simulink model "System_Template"  (R2021b)
settings: Solver=FixedStepDiscrete  StartTime=0.0  StopTime=0.001  FixedStep=1/312.5e6  RelTol=1e-3
undefined symbols (not defined in the file or in its folder): sigbuilder_block
settings Model: DataTypeOverride=Off  Creator=max_d  LastModifiedBy=max_d
settings SolverCC: AlgebraicLoopSolver=TrustRegion
settings DataIOCC: LimitDataPoints=on  SaveOutput=off  SaveTime=off
settings OptimizationCC: BlockReduction=off  ConditionallyExecuteInputs=off  DefaultParameterBehavior=Inlined  LifeSpan=inf
settings DebuggingCC: AlgebraicLoopMsg=error  SingleTaskRateTransMsg=error  AllowSymbolicDim=off  StrictBusMsg=ErrorOnBusTreatedAsVector  SFUnexpectedBacktrackingDiag=warning  SFNoUnconditionalDefaultTransitionDiag=warning  SFExecutionAtInitializationDiag=none  SFMachineParentedDataDiag=warning  ArithmeticOperatorsInVariantConditions=warning
settings HardwareCC: ProdBitPerPointer=32  ProdBitPerSizeT=32  ProdBitPerPtrDiffT=32  ProdLargestAtomicFloat=None  ProdIntDivRoundTo=Undefined  ProdEndianess=Unspecified  ProdWordSize=32  ProdHWDeviceType=ASIC/FPGA->ASIC/FPGA  ProdEqTarget=off
settings SFSimCC: SimUseLocalCustomCode=off  CustomCodeUndefinedFunction=UseInterfaceOnly
settings RTWCC: RTWUseLocalCustomCode=off
settings CodeAppCC: StateflowObjectComments=on
settings GRTTargetCC: TargetLangStandard=C89/C90 (ANSI)
settings ConfigComp: CovScope=ReferencedModels  CovMetricSettings=dw  CovSaveCumulativeToWorkspaceVar=on  CovSaveSingleToWorkspaceVar=on  CovExternalEMLEnable=off  CovSFcnEnable=off

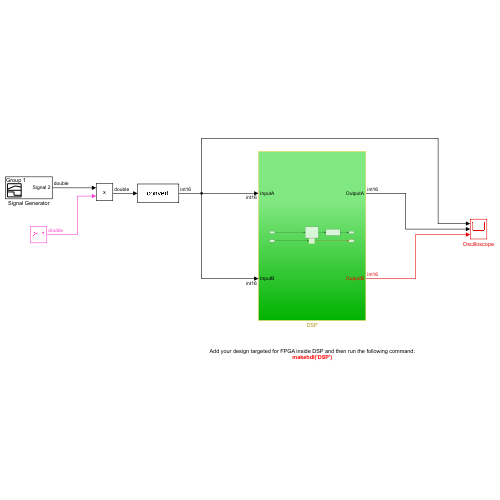
[thumbnail: Simulink's stored preview of the top-level diagram]
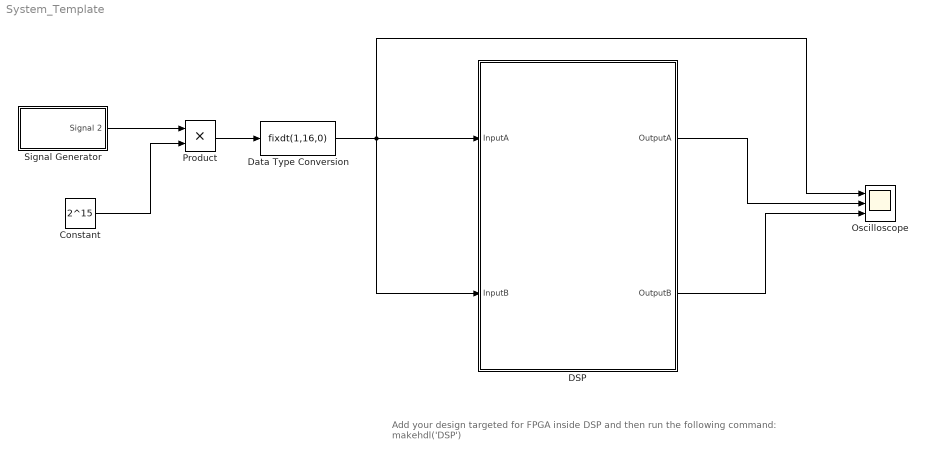
== system System_Template ==
  note: Add your design targeted for FPGA inside DSP and then run the following command:
      | makehdl('DSP')
  Constant : Constant  Value=2^15
  DSP : Subsystem
  Data Type Conversion : DataTypeConversion  OutDataTypeStr=fixdt(1,16,0)
  Oscilloscope : Scope  NumInputPorts=3
  Product : Product
  Signal Generator : Subsystem  Tag=STV Subsys  LoadFcn=sigbuilder_block('load');  StartFcn=sigbuilder_block('start');  StopFcn=sigbuilder_block('stop');  ClipboardFcn=sigbuilder_block('clipboard');  mask(Sigbuilder block){tuvar=[0:10]}
      mask help: Simulink:masks:SigbuilderBlock_MD
      mask init:
      | if ~strcmp(get_param(bdroot(gcbh),'SimulationStatus'),'stopped') tuvar = sigbuilder_block('maskInit'); end
      settings: CopyFcn=sigbuilder_block('copy');  DeleteFcn=sigbuilder_block('delete');  ModelCloseFcn=sigbuilder_block('modelClose');  PreSaveFcn=sigbuilder_block('preSave');  PauseFcn=sigbuilder_block('pause');  ContinueFcn=sigbuilder_block('continue');  NameChangeFcn=sigbuilder_block('namechange');  OpenFcn=sigbuilder_block('open',[437.25 199.5 550.5 399.75 ]);  CloseFcn=sigbuilder_block('close');
      mask Display: plot(0, 0, 100, 100,[2, 2, 32, 32, 2], [68, 8, 8, 68, 68],[32, 2], [38, 38], [32, 19, 2],[53, 60, 44], [32, 17, 17, 2],[16, 16, 31, 31]);txt = getActiveGroup(gcbh);text(2, 100, txt,'verticalAlignment', 'top');
  wires:
  DSP/1(OutputA) -> Oscilloscope/2
  DSP/2(OutputB) -> Oscilloscope/3
  Signal Generator/1(Signal 2) -> Product/1
  Constant/1 -> Product/2
  Product/1 -> Data Type Conversion/1
  Data Type Conversion/1 -> Oscilloscope/1, DSP/1(InputA), DSP/2(InputB)

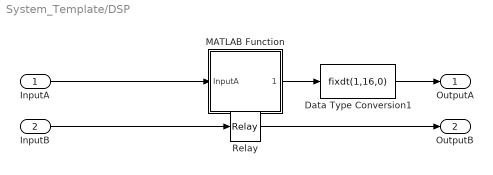
== system System_Template/DSP ==
  InputA : Inport  OutDataTypeStr=fixdt(1,16,0)
  InputB : Inport  Port=2  OutDataTypeStr=fixdt(1,16,0)
  Data Type Conversion1 : DataTypeConversion  OutDataTypeStr=fixdt(1,16,0)
  MATLAB Function : Subsystem  TreatAsAtomicUnit=on  Variant=on  VariantControlMode=label  VariantControl=Choice  LabelModeActiveChoice=(default)
  Relay : Relay  OnSwitchValue=floor(2^15/10)  OffSwitchValue=-floor(2^15/10)  OnOutputValue=2^15-1  OutDataTypeStr=fixdt(1,16,0)
  OutputA : Outport  OutDataTypeStr=fixdt(1,16,0)  VectorParamsAs1DForOutWhenUnconnected=off
  OutputB : Outport  Port=2  OutDataTypeStr=fixdt(1,16,0)  VectorParamsAs1DForOutWhenUnconnected=off
  wires:
  Data Type Conversion1/1 -> OutputA/1
  InputB/1 -> Relay/1
  Relay/1 -> OutputB/1
  InputA/1 -> MATLAB Function/1(InputA)
  MATLAB Function/1(OutputA) -> Data Type Conversion1/1

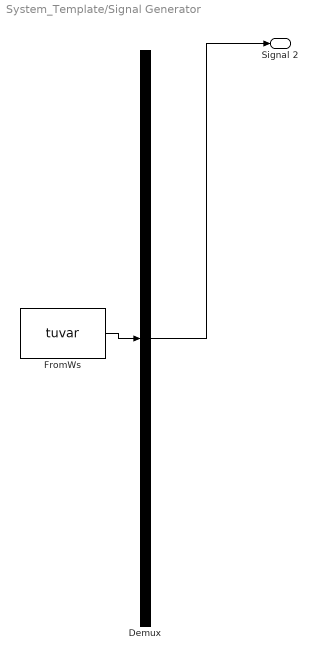
== system System_Template/Signal Generator ==
  Demux : Demux  Tag=STV Demux  Outputs=1
      settings: DisplayOption=none
  FromWs : FromWorkspace  Tag=STV FromWs  VariableName=tuvar
      SigBuilderData=|
      | common.afterFinalStr = 'Extrapolate'
      | common.sampleTime = 0
      | dataSet.timeRange = [0 0.001]
      | dataSet.name = 'Group 1'
      | sbobj.Groups.Name = 'Group 1'
      | sbobj.Groups.Signals.Name = 'Signal 2'
      | sbobj.Groups.Signals.XData = [0 2.5e-07 5e-07 7.5e-07 1e-06 1.25e-06 1.5e-06 1.75e-06 2e-06 2.25e-06 2.5e-06 2.75e-06 ... (4001 elements, 1x4001)]
      | sbobj.Groups.Signals.YData = [0.0343957315647 0.176356157537 0.0819524449776 0.0936305274591 -0.146970539233 0.105590892644 -0.128251371742 -0.039701741783 -0.00694007713759 0.070966955857 0.0238735264584 -0.0686801559142 ... (4001 elements, 1x4001)]
      | sbobj.Groups.TimeRange = [0 0.001]
  Signal 2 : Outport  Tag=STV Outport
  wires:
  FromWs/1 -> Demux/1
  Demux/1 -> Signal 2/1

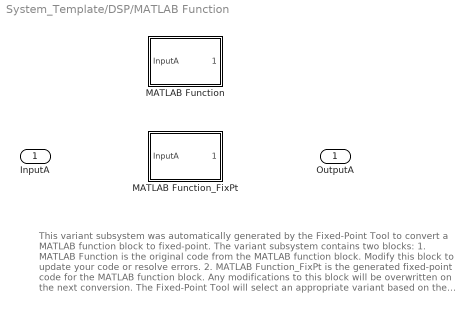
== system System_Template/DSP/MATLAB Function ==
  note: This variant subsystem was automatically generated by the Fixed-Point Tool to convert a MATLAB function block to fixed-point.
      |
      | The variant subsystem contains two blocks:
      | 1. MATLAB Function is the original code from the MATLAB function block. Modify this block to update your code or resolve errors.
      |
      | 2. MATLAB Function_FixPt is the generated fixed-point code for the MATLAB function block. Any modifications to this block will be overwritten on the next conversion.
      |
      | The Fixed-Point Tool will select an appropriate variant based on the Model Settings. Learn more. .
  InputA : Inport
  MATLAB Function : MATLAB Function  TreatAsAtomicUnit=on  VariantControl=false()
  MATLAB Function_FixPt : MATLAB Function  TreatAsAtomicUnit=on  VariantControl=(default)
  OutputA : Outport

== matlab function System_Template/DSP/MATLAB Function/MATLAB Function ==
  data: InputA input; OutputA output
function OutputA = Schimitt_Trigger(InputA)
%#codegen
persistent out0; %Retains variable value between function calls.
if isempty(out0) %Initialize the value for the first call.
    out0 = 0;
end

upperThreshold = floor(2^15/10); %Set the upper threshold to 1/10 of the full positive range.
lowerThreshold = -floor(2^15/10); %Set the lower threshold to 1/10 of the full negative range.
 
if InputA >upperThreshold %Logic to perform the Schmitt trigger function.
    out0 = 2^15-1; %Map to the highest positive number.
elseif InputA <lowerThreshold
    out0 = 0;
end

OutputA = out0; %Assign variable out0 to OutputA.

== matlab function System_Template/DSP/MATLAB Function/MATLAB Function_FixPt ==
  settings: fimath=fimath('RoundingMethod', 'Floor', 'OverflowAction', 'Wrap', 'ProductMode', 'FullPrecision', 'MaxProductWordLength', 128, 'SumMode', 'FullPrecision', 'MaxSumWordLength', 128)
  data: InputA input; OutputA output
%auto-generated
function OutputA = Schimitt_Trigger_fixpt(InputA)
%#codegen
fm = get_fimath();
InputA = fi(InputA, 1, 16, 1, fm);

persistent out0; %Retains variable value between function calls.
if isempty(out0) %Initialize the value for the first call.
    out0 = fi(0, 0, 16, 0, fm);
end

upperThreshold = fi(floor(2^15/10), 0, 16, 4, fm); %Set the upper threshold to 1/10 of the full positive range.
lowerThreshold = fi(-floor(2^15/10), 1, 16, 3, fm); %Set the lower threshold to 1/10 of the full negative range.
 
if InputA >upperThreshold %Logic to perform the Schmitt trigger function.
    out0(:) = 2^15-1; %Map to the highest positive number.
elseif InputA <lowerThreshold
    out0(:) = 0;
end

OutputA = fi(out0, 0, 16, 0, fm); %Assign variable out0 to OutputA.
end


function fm = get_fimath()
	fm = fimath('RoundingMethod', 'Floor',...
	     'OverflowAction', 'Wrap',...
	     'ProductMode','FullPrecision',...
	     'MaxProductWordLength', 128,...
	     'SumMode','FullPrecision',...
	     'MaxSumWordLength', 128);
end
